simulink model "PMSM"  (R2018b)
settings: Solver=VariableStepAuto  StartTime=0.0  StopTime=tmax  RelTol=1e-3
values from neighbouring files (symbols this model uses):
  J = 10    [RunPMSM.m]
  kp = 100    [RunPMSM.m]
  kpw = 100    [RunPMSM.m]
  L1d = 1e-4    (= 0.0001)    [RunPMSM.m]
  L1q = 1e-3    (= 0.001)    [RunPMSM.m]
  p = 1    [RunPMSM.m]
  psi = 10    [RunPMSM.m]
  R1 = 10    [RunPMSM.m]
settings Model: Creator=raphael  LastModifiedBy=raphael

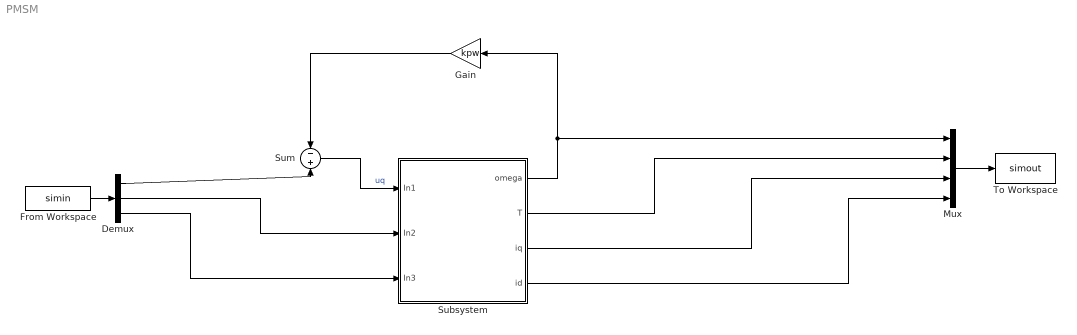
== system PMSM ==
  Demux : Demux  Outputs=3
  From Workspace : FromWorkspace  VariableName=simin  SampleTime=0
  Gain : Gain  Gain=kpw
  Mux : Mux
  Subsystem : Subsystem
  Sum : Sum  Inputs=-+
  To Workspace : ToWorkspace  VariableName=simout  SaveFormat=Timeseries  SampleTime=-1
  wires:
  From Workspace/1 -> Demux/1
  Mux/1 -> To Workspace/1
  Demux/2 -> Subsystem/2(In2)
  Demux/3 -> Subsystem/3(In3)
  Subsystem/1(omega) -> Gain/1, Mux/1
  Subsystem/2(T) -> Mux/2
  Subsystem/3(iq) -> Mux/3
  Subsystem/4(id) -> Mux/4
  Sum/1 -> Subsystem/1(In1)  "uq"
  Demux/1 -> Sum/2
  Gain/1 -> Sum/1

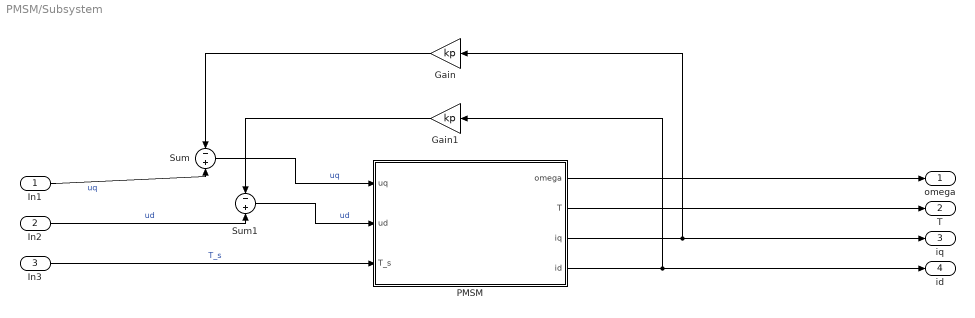
== system PMSM/Subsystem ==
  In1 : Inport
  In2 : Inport  Port=2
  In3 : Inport  Port=3
  Gain : Gain  Gain=kp
  Gain1 : Gain  Gain=kp
  PMSM : Subsystem
  Sum : Sum  Inputs=-+
  Sum1 : Sum  Inputs=-+
  omega : Outport
  T : Outport  Port=2
  iq : Outport  Port=3
  id : Outport  Port=4
  wires:
  Sum/1 -> PMSM/1(uq)  "uq"
  Sum1/1 -> PMSM/2(ud)  "ud"
  In3/1 -> PMSM/3(T_s)  "T_s"
  PMSM/1(omega) -> omega/1
  PMSM/2(T) -> T/1
  PMSM/3(iq) -> Gain/1, iq/1
  PMSM/4(id) -> Gain1/1, id/1
  In1/1 -> Sum/2  "uq"
  Gain/1 -> Sum/1
  In2/1 -> Sum1/2  "ud"
  Gain1/1 -> Sum1/1

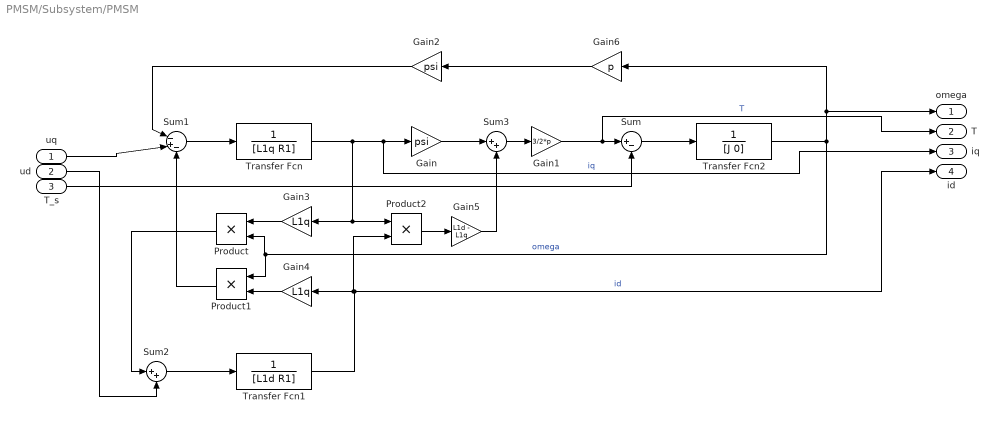
== system PMSM/Subsystem/PMSM ==
  uq : Inport
  ud : Inport  Port=2
  T_s : Inport  Port=3
  Gain : Gain  Gain=psi
  Gain1 : Gain  Gain=3/2*p
  Gain2 : Gain  Gain=psi
  Gain3 : Gain  Gain=L1q
  Gain4 : Gain  Gain=L1q
  Gain5 : Gain  Gain=L1d - L1q
  Gain6 : Gain  Gain=p
  Product : Product
  Product1 : Product
  Product2 : Product
  Sum : Sum  Inputs=|+-
  Sum1 : Sum  Inputs=|-+-
  Sum2 : Sum  Inputs=|++
  Sum3 : Sum  Inputs=|++
  Transfer Fcn : TransferFcn  Denominator=[L1q R1]
  Transfer Fcn1 : TransferFcn  Denominator=[L1d R1]
  Transfer Fcn2 : TransferFcn  Denominator=[J 0]
  omega : Outport
  T : Outport  Port=2
  iq : Outport  Port=3
  id : Outport  Port=4
  wires:
  ud/1 -> Sum2/2
  Product2/1 -> Gain5/1
  Sum/1 -> Transfer Fcn2/1
  Gain5/1 -> Sum3/2
  Product/1 -> Sum2/1
  Sum2/1 -> Transfer Fcn1/1
  Sum3/1 -> Gain1/1
  Gain/1 -> Sum3/1
  Gain6/1 -> Gain2/1
  Product1/1 -> Sum1/3
  Gain4/1 -> Product1/2
  Gain3/1 -> Product/1
  Gain2/1 -> Sum1/1
  Transfer Fcn2/1 -> Product1/1, Product/2, omega/1, Gain6/1  "omega"
  Transfer Fcn/1 -> Product2/1, Gain3/1, iq/1, Gain/1  "iq"
  Gain1/1 -> T/1, Sum/1  "T"
  T_s/1 -> Sum/2
  uq/1 -> Sum1/2
  Sum1/1 -> Transfer Fcn/1
  Transfer Fcn1/1 -> id/1, Product2/2, Gain4/1  "id"
